simulink model "PID_motor"  (R2019b)
settings: Solver=VariableStepAuto  StartTime=0.0  StopTime=30  RelTol=1e-3
PreLoadFcn:
  | load('task1_20.m')
values from neighbouring files (symbols this model uses):
  b = 6.797e-04    (= 0.0006797)    [task1_20.m]
  J = 0.007    [task1_20.m]
  ke = 0.2154    [task1_20.m]
  kt = 0.1186    [task1_20.m]
  L = 0    [task1_20.m]
  Nf = 100    [task1_20.m]
  R = 2.400    (= 2.4)    [task1_20.m]
settings Model: Creator=Ommie  LastModifiedBy=Ommie

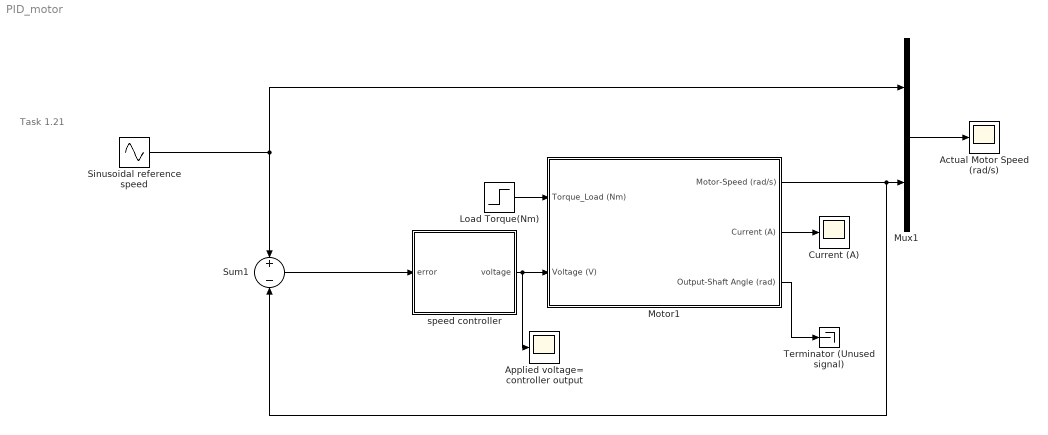
== system PID_motor ==
  note: Task 1.21
  Actual Motor Speed (rad/s) : Scope
  "Applied voltage= controller output " : Scope
  Current (A) : Scope
  Load Torque(Nm) : Step  Time=15  After=0.25  SampleTime=0
  Motor1 : Subsystem
  Mux1 : Mux  Inputs=2
  Sinusoidal reference speed : Sin  Amplitude=5  Bias=15  SampleTime=0
  Sum1 : Sum  Inputs=+|-
  Terminator (Unused signal) : Terminator
  speed controller : Subsystem
  wires:
  speed controller/1(voltage) -> "Applied voltage= controller output "/1, Motor1/2(Voltage (V))
  Motor1/1(Motor-Speed (rad/s)) -> Sum1/2, Mux1/2
  Sinusoidal reference speed/1 -> Mux1/1, Sum1/1
  Mux1/1 -> Actual Motor Speed (rad/s)/1
  Motor1/3(Output-Shaft Angle (rad)) -> Terminator (Unused signal)/1
  Load Torque(Nm)/1 -> Motor1/1(Torque_Load (Nm))
  Sum1/1 -> speed controller/1(error)
  Motor1/2(Current (A)) -> Current (A)/1

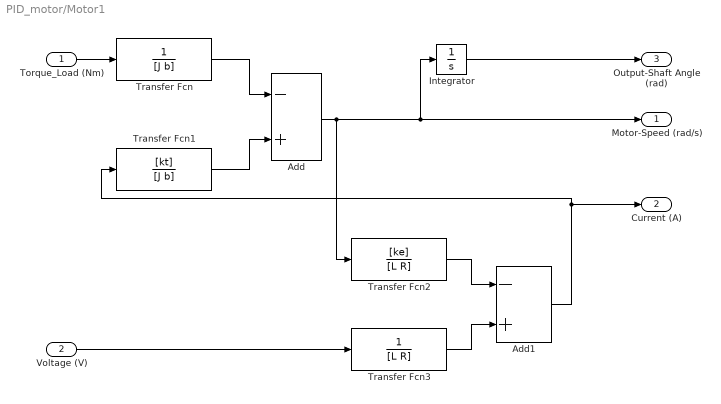
== system PID_motor/Motor1 ==
  Torque_Load (Nm) : Inport
  Voltage (V) : Inport  Port=2
  Add : Sum  Inputs=-+
  Add1 : Sum  Inputs=-+
  Integrator : Integrator
  Transfer Fcn : TransferFcn  Denominator=[J b]
  Transfer Fcn1 : TransferFcn  Numerator=[kt]  Denominator=[J b]
  Transfer Fcn2 : TransferFcn  Numerator=[ke]  Denominator=[L R]
  Transfer Fcn3 : TransferFcn  Numerator=1  Denominator=[L R]
  Motor-Speed (rad/s) : Outport  VectorParamsAs1DForOutWhenUnconnected=off
  Current (A) : Outport  Port=2  VectorParamsAs1DForOutWhenUnconnected=off
  Output-Shaft Angle (rad) : Outport  Port=3  VectorParamsAs1DForOutWhenUnconnected=off
  wires:
  Add1/1 -> Current (A)/1, Transfer Fcn1/1
  Torque_Load (Nm)/1 -> Transfer Fcn/1
  Transfer Fcn1/1 -> Add/2
  Integrator/1 -> Output-Shaft Angle (rad)/1
  Voltage (V)/1 -> Transfer Fcn3/1
  Transfer Fcn/1 -> Add/1
  Transfer Fcn2/1 -> Add1/1
  Transfer Fcn3/1 -> Add1/2
  Add/1 -> Motor-Speed (rad/s)/1, Integrator/1, Transfer Fcn2/1

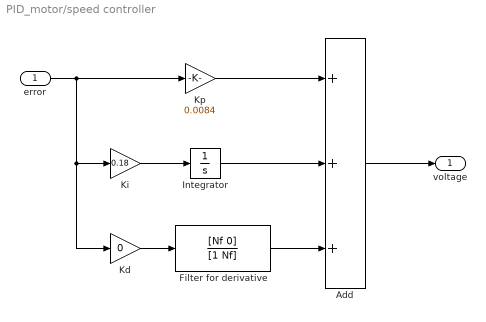
== system PID_motor/speed controller ==
  error : Inport
  Add : Sum  Inputs=+++
  Filter for derivative : TransferFcn  Numerator=[Nf 0]  Denominator=[1 Nf]
  Integrator : Integrator
  Kd : Gain  Gain=0
  Ki : Gain  Gain=0.18
  Kp : Gain  Gain=0.0084
  voltage : Outport  VectorParamsAs1DForOutWhenUnconnected=off
  wires:
  Filter for derivative/1 -> Add/3
  Kp/1 -> Add/1
  Integrator/1 -> Add/2
  error/1 -> Kd/1, Ki/1, Kp/1
  Add/1 -> voltage/1
  Ki/1 -> Integrator/1
  Kd/1 -> Filter for derivative/1
